simulink model "Model_Masina"  (R2021b)
settings: Solver=ode45  StartTime=0.0  StopTime=10  FixedStep=0.01  RelTol=1e-3
values from neighbouring files (symbols this model uses):
  AirDensity_kgpm3 = 1.225    [vehicle_controller.mat]
  BatteryCapacity_Wh = 83    [vehicle_controller.mat]
  BatteryInitialEnergy = 58.1    [vehicle_controller.mat]
  BatteryMaxVoltage_V = 96    [vehicle_controller.mat]
  BatteryVoltageCoefficient_x = [0 0.1 0.2 0.3 0.4 0.5 0.6 0.7 0.8 0.9 1]    [vehicle_controller.mat]
  BatteryVoltageCoefficient_y = [0.833333333333 0.85 0.866666666667 0.883333333333 0.9 0.916666666667 0.933333333333 0.95 0.966666666667 0.983333333333 1]    [vehicle_controller.mat]
  BodyInitialSpeed_mps = 0    [vehicle_controller.mat]
  BodyMass_kg = 900    [vehicle_controller.mat]
  CombustionEngineMaxTorque_Nm = 100    [vehicle_controller.mat]
  DragArea_m2 = 4.5    [vehicle_controller.mat]
  DragCoeficient_1 = 0.4    [vehicle_controller.mat]
  FrictionCoefficient_Nsprad = 0.01    [vehicle_controller.mat]
  GearboxRatio_0_1 = 3    [vehicle_controller.mat]
  Ke = 0.1178    [vehicle_controller.mat]
  Kt = 0.668    [vehicle_controller.mat]
  L = looptransfer.Lo    [H_infinity_control_design.m]    (also in LoopShaping.m = G*K; Vehicle_Car_Controller.m = P * C)
  R = 0.141176    [vehicle_controller.mat]
  WheelDiameter_m = 0.5    [vehicle_controller.mat]
libraries: simulink x2, simulink_extras x1
settings Model: Creator=matti  LastModifiedBy=beni
settings DataIOCC: ReturnWorkspaceOutputs=off
settings DebuggingCC: SFMachineParentedDataDiag=warning

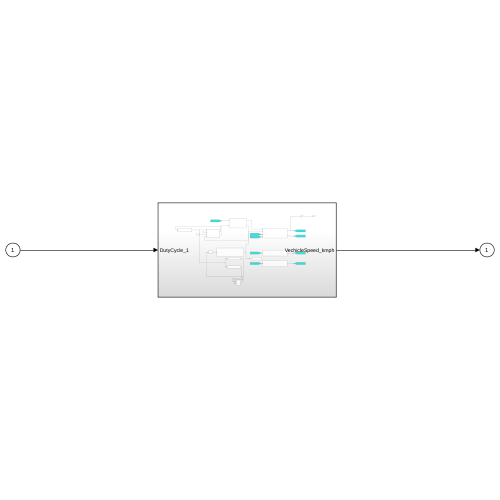
[thumbnail: Simulink's stored preview of the top-level diagram]
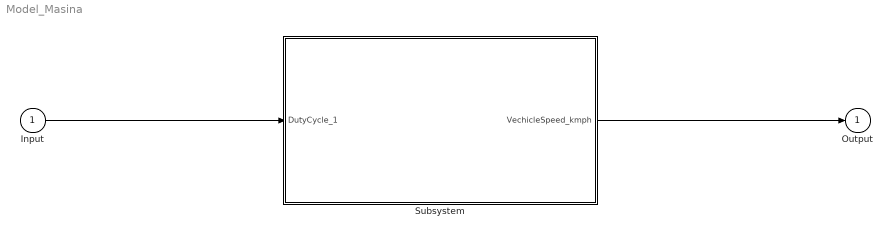
== system Model_Masina ==
  Input : Inport
  Subsystem : Subsystem
  Output : Outport
  wires:
  Input/1 -> Subsystem/1(DutyCycle_1)
  Subsystem/1(VechicleSpeed_kmph) -> Output/1

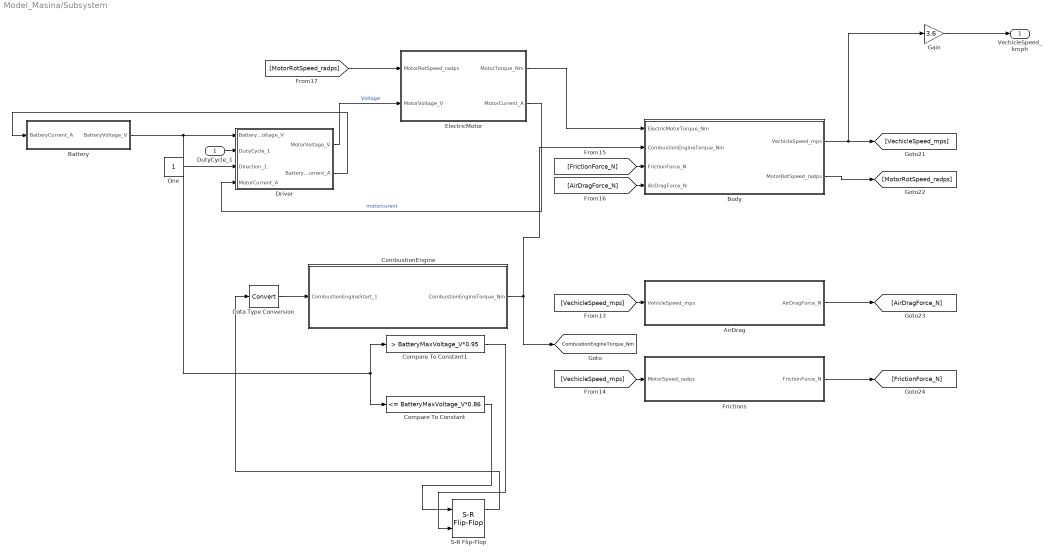
== system Model_Masina/Subsystem ==
  DutyCycle_1 : Inport
  AirDrag : Subsystem
  Battery : Subsystem
  Body : Subsystem
  CombustionEngine : Subsystem
  Compare To Constant : simulink/Logic and Bit Operations/Compare To Constant  relop=<=  const=BatteryMaxVoltage_V*0.86  OutDataTypeStr=boolean
  Compare To Constant1 : simulink/Logic and Bit Operations/Compare To Constant  relop=>  const=BatteryMaxVoltage_V*0.95  OutDataTypeStr=boolean
  Data Type Conversion : DataTypeConversion
  Driver : Subsystem
  ElectricMotor : Subsystem
  Frictions : Subsystem
  Gain : Gain  Gain=3.6
  One : Constant  OutDataTypeStr=Inherit: Inherit via back propagation
  S-R Flip-Flop : simulink_extras/Flip Flops/S-R Flip-Flop  initial_condition=0
  VechicleSpeed_kmph : Outport
  tag scope: CombustionEngineTorque_Nm=global
  wires:
  One/1 -> Driver/3(Direction_1)
  ElectricMotor/1(MotorTorque_Nm) -> Body/1(ElectricMotorTorque_Nm)
  [FrictionForce_N] -> Body/3(FrictionForce_N)
  Body/1(VechicleSpeed_mps) -> [VechicleSpeed_mps], Gain/1
  Body/2(MotorRotSpeed_radps) -> [MotorRotSpeed_radps]
  AirDrag/1(AirDragForce_N) -> [AirDragForce_N]
  Frictions/1(FrictionForce_N) -> [FrictionForce_N]
  [VechicleSpeed_mps] -> AirDrag/1(VehicleSpeed_mps)
  [AirDragForce_N] -> Body/4(AirDragForce_N)
  [MotorRotSpeed_radps] -> ElectricMotor/1(MotorRotSpeed_radps)
  [VechicleSpeed_mps] -> Frictions/1(MotorSpeed_radps)
  ElectricMotor/2(MotorCurrent_A) -> Driver/4(MotorCurrent_A)  "motorcurent"
  DutyCycle_1/1 -> Driver/2(DutyCycle_1)
  Gain/1 -> VechicleSpeed_kmph/1
  Data Type Conversion/1 -> CombustionEngine/1(CombustionEngineStart_1)
  CombustionEngine/1(CombustionEngineTorque_Nm) -> Body/2(CombustionEngineTorque_Nm), [CombustionEngineTorque_Nm]
  Driver/2(BatteryCurrent_A) -> Battery/1(BatteryCurrent_A)
  Driver/1(MotorVoltage_V) -> ElectricMotor/2(MotorVoltage_V)  "Voltage"
  Compare To Constant1/1 -> S-R Flip-Flop/2
  Compare To Constant/1 -> S-R Flip-Flop/1
  S-R Flip-Flop/1 -> Data Type Conversion/1
  Battery/1(BatteryVoltage_V) -> Driver/1(BatteryVoltage_V), Compare To Constant1/1, Compare To Constant/1

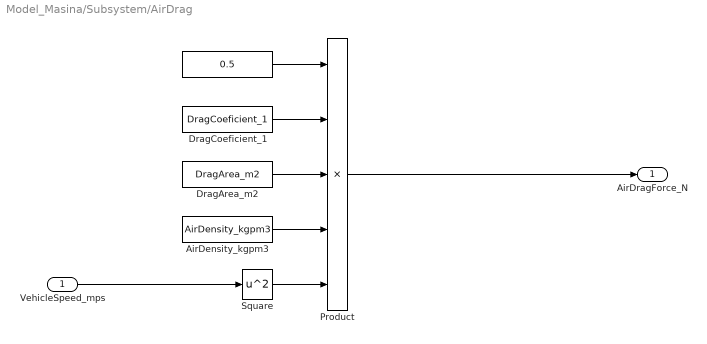
== system Model_Masina/Subsystem/AirDrag ==
  VehicleSpeed_mps : Inport
  " " : Constant  Value=0.5
  AirDensity_kgpm3 : Constant  Value=AirDensity_kgpm3
  DragArea_m2 : Constant  Value=DragArea_m2
  DragCoeficient_1 : Constant  Value=DragCoeficient_1
  Product : Product  Inputs=5
  Square : Math  Operator=square  SaturateOnIntegerOverflow=on
  AirDragForce_N : Outport
  wires:
  VehicleSpeed_mps/1 -> Square/1
  Square/1 -> Product/5
  DragArea_m2/1 -> Product/3
  AirDensity_kgpm3/1 -> Product/4
  DragCoeficient_1/1 -> Product/2
  " "/1 -> Product/1
  Product/1 -> AirDragForce_N/1

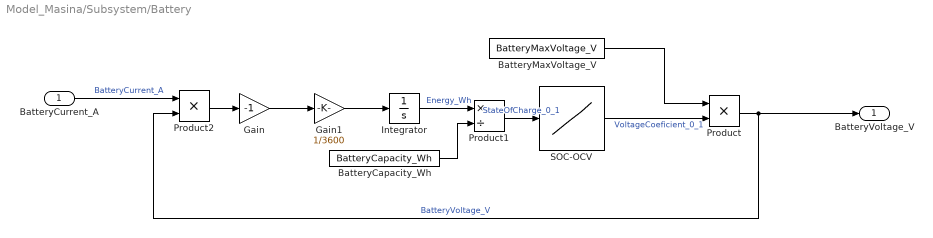
== system Model_Masina/Subsystem/Battery ==
  BatteryCurrent_A : Inport
  BatteryCapacity_Wh : Constant  Value=BatteryCapacity_Wh
  BatteryMaxVoltage_V : Constant  Value=BatteryMaxVoltage_V
  Gain : Gain  Gain=-1
  Gain1 : Gain  Gain=1/3600
  Integrator : Integrator  InitialCondition=BatteryInitialEnergy
  Product : Product
  Product1 : Product  Inputs=*/
  Product2 : Product
  SOC-OCV : Lookup_n-D  NumberOfTableDimensions=1  BreakpointsForDimension1=BatteryVoltageCoefficient_x  Table=BatteryVoltageCoefficient_y  InternalRulePriority=Speed  RndMeth=Simplest  InputSameDT=on
  BatteryVoltage_V : Outport
  wires:
  BatteryCurrent_A/1 -> Product2/1  "BatteryCurrent_A"
  Product/1 -> Product2/2, BatteryVoltage_V/1  "BatteryVoltage_V"
  Integrator/1 -> Product1/1  "Energy_Wh"
  SOC-OCV/1 -> Product/2  "VoltageCoeficient_0_1"
  BatteryMaxVoltage_V/1 -> Product/1
  BatteryCapacity_Wh/1 -> Product1/2
  Product1/1 -> SOC-OCV/1  "StateOfCharge_0_1"
  Product2/1 -> Gain/1
  Gain/1 -> Gain1/1
  Gain1/1 -> Integrator/1

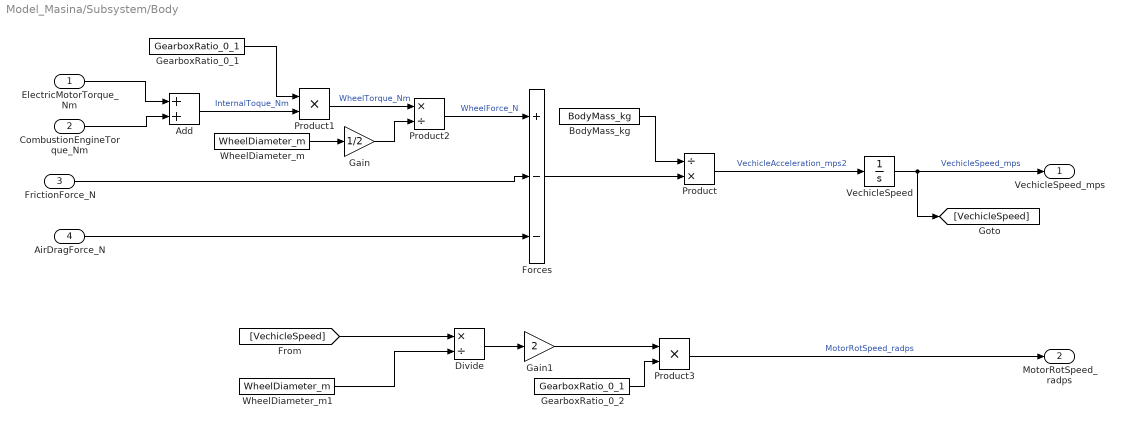
== system Model_Masina/Subsystem/Body ==
  ElectricMotorTorque_Nm : Inport
  CombustionEngineTorque_Nm : Inport  Port=2
  FrictionForce_N : Inport  Port=3
  AirDragForce_N : Inport  Port=4
  Add : Sum
  BodyMass_kg : Constant  Value=BodyMass_kg
  Divide : Product  Inputs=*/
  Forces : Sum  Inputs=+--
  Gain : Gain  Gain=1/2
  Gain1 : Gain  Gain=2
  GearboxRatio_0_1 : Constant  Value=GearboxRatio_0_1
  GearboxRatio_0_2 : Constant  Value=GearboxRatio_0_1
  Product : Product  Inputs=/*
  Product1 : Product
  Product2 : Product  Inputs=*/
  Product3 : Product  Inputs=**
  VechicleSpeed : Integrator  InitialCondition=BodyInitialSpeed_mps
  WheelDiameter_m : Constant  Value=WheelDiameter_m
  WheelDiameter_m1 : Constant  Value=WheelDiameter_m
  VechicleSpeed_mps : Outport
  MotorRotSpeed_radps : Outport  Port=2
  wires:
  VechicleSpeed/1 -> [VechicleSpeed], VechicleSpeed_mps/1  "VechicleSpeed_mps"
  Product/1 -> VechicleSpeed/1  "VechicleAcceleration_mps2"
  BodyMass_kg/1 -> Product/1
  Forces/1 -> Product/2
  AirDragForce_N/1 -> Forces/3
  FrictionForce_N/1 -> Forces/2
  ElectricMotorTorque_Nm/1 -> Add/1
  CombustionEngineTorque_Nm/1 -> Add/2
  Add/1 -> Product1/2  "InternalToque_Nm"
  GearboxRatio_0_1/1 -> Product1/1
  Product1/1 -> Product2/1  "WheelTorque_Nm"
  WheelDiameter_m/1 -> Gain/1
  Product2/1 -> Forces/1  "WheelForce_N"
  Gain/1 -> Product2/2
  [VechicleSpeed] -> Divide/1
  WheelDiameter_m1/1 -> Divide/2
  Divide/1 -> Gain1/1
  Gain1/1 -> Product3/1
  GearboxRatio_0_2/1 -> Product3/2
  Product3/1 -> MotorRotSpeed_radps/1  "MotorRotSpeed_radps"

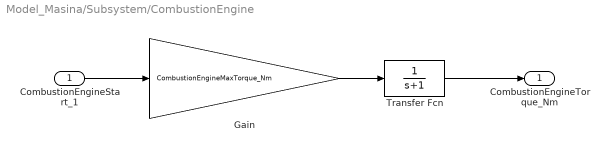
== system Model_Masina/Subsystem/CombustionEngine ==
  CombustionEngineStart_1 : Inport
  Gain : Gain  Gain=CombustionEngineMaxTorque_Nm
  Transfer Fcn : TransferFcn  Denominator=[1 1]
  CombustionEngineTorque_Nm : Outport
  wires:
  Transfer Fcn/1 -> CombustionEngineTorque_Nm/1
  CombustionEngineStart_1/1 -> Gain/1
  Gain/1 -> Transfer Fcn/1

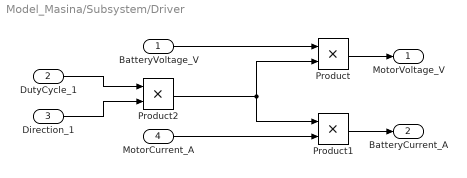
== system Model_Masina/Subsystem/Driver ==
  BatteryVoltage_V : Inport
  DutyCycle_1 : Inport  Port=2
  Direction_1 : Inport  Port=3
  MotorCurrent_A : Inport  Port=4
  Product : Product
  Product1 : Product
  Product2 : Product
  MotorVoltage_V : Outport
  BatteryCurrent_A : Outport  Port=2
  wires:
  BatteryVoltage_V/1 -> Product/1
  Product/1 -> MotorVoltage_V/1
  Product2/1 -> Product1/1, Product/2
  MotorCurrent_A/1 -> Product1/2
  Product1/1 -> BatteryCurrent_A/1
  DutyCycle_1/1 -> Product2/1
  Direction_1/1 -> Product2/2

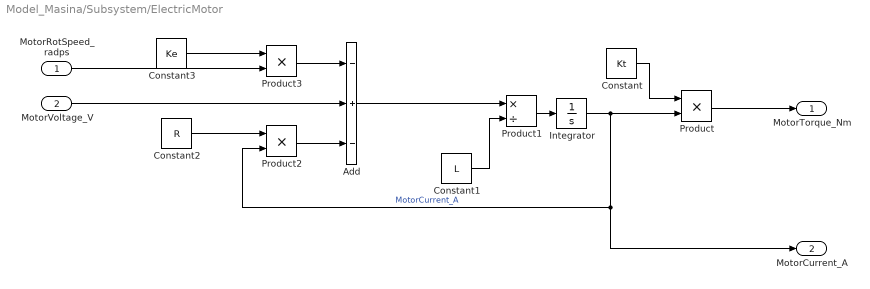
== system Model_Masina/Subsystem/ElectricMotor ==
  MotorRotSpeed_radps : Inport
  MotorVoltage_V : Inport  Port=2
  Add : Sum  Inputs=-+-
  Constant : Constant  Value=Kt
  Constant1 : Constant  Value=L
  Constant2 : Constant  Value=R
  Constant3 : Constant  Value=Ke
  Integrator : Integrator
  Product : Product
  Product1 : Product  Inputs=*/
  Product2 : Product
  Product3 : Product
  MotorTorque_Nm : Outport
  MotorCurrent_A : Outport  Port=2
  wires:
  Product/1 -> MotorTorque_Nm/1
  Integrator/1 -> Product2/2, MotorCurrent_A/1, Product/2  "MotorCurrent_A"
  Constant/1 -> Product/1
  Product1/1 -> Integrator/1
  Constant1/1 -> Product1/2
  Add/1 -> Product1/1
  Product2/1 -> Add/3
  Constant2/1 -> Product2/1
  MotorVoltage_V/1 -> Add/2
  Constant3/1 -> Product3/1
  Product3/1 -> Add/1
  MotorRotSpeed_radps/1 -> Product3/2

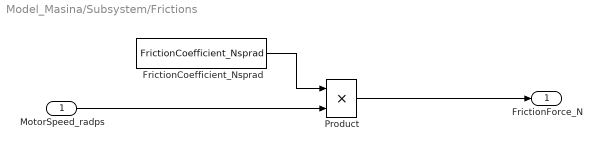
== system Model_Masina/Subsystem/Frictions ==
  MotorSpeed_radps : Inport
  FrictionCoefficient_Nsprad : Constant  Value=FrictionCoefficient_Nsprad
  Product : Product
  FrictionForce_N : Outport
  wires:
  Product/1 -> FrictionForce_N/1
  MotorSpeed_radps/1 -> Product/2
  FrictionCoefficient_Nsprad/1 -> Product/1
